simulink model "Valenton_JJ_MATLAB_No2_REDUCED"  (R2023b)
settings: Solver=VariableStepAuto  StartTime=0.0  StopTime=10.0  RelTol=1e-3
settings Model: Creator=ACER  LastModifiedBy=ACER

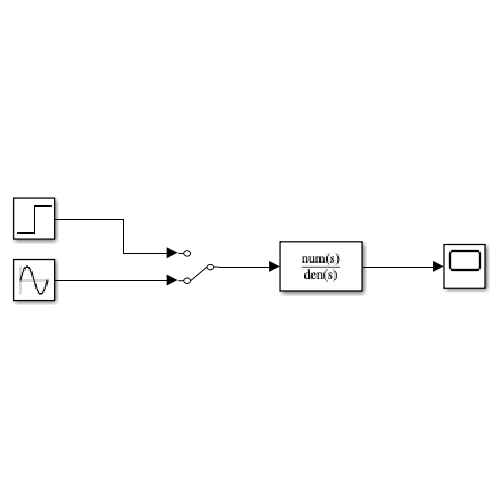
[thumbnail: Simulink's stored preview of the top-level diagram]
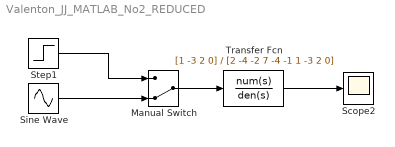
== system Valenton_JJ_MATLAB_No2_REDUCED ==
  Manual Switch : ManualSwitch  CurrentSetting=0
  Scope2 : Scope
  Sine Wave : Sin  SampleTime=0
  Step1 : Step  SampleTime=0
  Transfer Fcn : TransferFcn  Numerator=[1 -3 2 0]  Denominator=[2 -4 -2 7 -4 -1 1 -3 2 0]
  wires:
  Step1/1 -> Manual Switch/1
  Manual Switch/1 -> Transfer Fcn/1
  Sine Wave/1 -> Manual Switch/2
  Transfer Fcn/1 -> Scope2/1
